simulink model "MPC_MG_freq_27072022"  (R2021b)
settings: Solver=VariableStepAuto  StartTime=0.0  StopTime=10  RelTol=1e-3
model workspace (MAT data in the model file):
  Ts : Simulink.Parameter (value not decoded)
  secondary_on : Simulink.Parameter (value not decoded)
values from neighbouring files (symbols this model uses):
  A = zeros(4,4)    [MPC_MG_script_raw_dmpc.m]    (also in MPG_MG_July.m = [0 1 1 1; 1 0 0 0; 1 0 0 0; 1 0 0 0]; MPG_MG_freq_script.m = ones(4) - eye(4); Script.m = [0 1 1 1 ; 1 0 1 1 ; 1 1 0 1 ; 1 1 1 0])
  a12 = 0    [Four_DG_MG_PrimaryOnlyScript.m]    (also in MPC_MG_script_raw_dmpc.m; MPC_MG_secondary_script.m)
  a14 = 0    [Four_DG_MG_PrimaryOnlyScript.m]    (also in MPC_MG_script_raw_dmpc.m; MPC_MG_secondary_script.m)
  a21 = 1    [Four_DG_MG_PrimaryOnlyScript.m]    (also in MPC_MG_script_raw_dmpc.m; MPC_MG_secondary_script.m)
  a23 = 0    [Four_DG_MG_PrimaryOnlyScript.m]    (also in MPC_MG_script_raw_dmpc.m; MPC_MG_secondary_script.m)
  a32 = 1    [Four_DG_MG_PrimaryOnlyScript.m]    (also in MPC_MG_script_raw_dmpc.m; MPC_MG_secondary_script.m)
  a34 = 0    [Four_DG_MG_PrimaryOnlyScript.m]    (also in MPC_MG_script_raw_dmpc.m; MPC_MG_secondary_script.m)
  a41 = 1    [Four_DG_MG_PrimaryOnlyScript.m]    (also in MPC_MG_script_raw_dmpc.m; MPC_MG_secondary_script.m)
  a43 = 0    [Four_DG_MG_PrimaryOnlyScript.m]    (also in MPC_MG_script_raw_dmpc.m; MPC_MG_secondary_script.m)
  b1v = 1    [Four_DG_MG_PrimaryOnlyScript.m]    (also in MPC_MG_script_raw_dmpc.m; MPC_MG_secondary_script.m; MPG_MG_July.m; MPG_MG_freq_script.m)
  b1w = 1    [Four_DG_MG_PrimaryOnlyScript.m]    (also in MPC_MG_script_raw_dmpc.m; MPC_MG_secondary_script.m; MPG_MG_July.m; MPG_MG_freq_script.m)
  b2v = 0    [Four_DG_MG_PrimaryOnlyScript.m]    (also in MPC_MG_script_raw_dmpc.m; MPC_MG_secondary_script.m; MPG_MG_July.m; MPG_MG_freq_script.m)
  b2w = 0    [Four_DG_MG_PrimaryOnlyScript.m]    (also in MPC_MG_script_raw_dmpc.m; MPC_MG_secondary_script.m; MPG_MG_July.m; MPG_MG_freq_script.m)
  b3v = 0    [Four_DG_MG_PrimaryOnlyScript.m]    (also in MPC_MG_script_raw_dmpc.m; MPC_MG_secondary_script.m; MPG_MG_July.m; MPG_MG_freq_script.m)
  b3w = 0    [Four_DG_MG_PrimaryOnlyScript.m]    (also in MPC_MG_script_raw_dmpc.m; MPC_MG_secondary_script.m; MPG_MG_July.m; MPG_MG_freq_script.m)
  b4v = 0    [Four_DG_MG_PrimaryOnlyScript.m]    (also in MPC_MG_script_raw_dmpc.m; MPC_MG_secondary_script.m; MPG_MG_July.m; MPG_MG_freq_script.m)
  b4w = 0    [Four_DG_MG_PrimaryOnlyScript.m]    (also in MPC_MG_script_raw_dmpc.m; MPC_MG_secondary_script.m; MPG_MG_July.m; MPG_MG_freq_script.m)
  C_f = 50e-6    (= 5e-05)    [Four_DG_MG_PrimaryOnlyScript.m]    (also in MPC_MG_script.m; MPC_MG_script_raw_dmpc.m; MPC_MG_secondary_script.m; MPG_MG_July.m)
  cf = 60    [Four_DG_MG_PrimaryOnlyScript.m]    (also in MPC_MG_script_raw_dmpc.m = 40; MPC_MG_secondary_script.m = 40; MPG_MG_July.m = 100; MPG_MG_freq_script.m = 100)
  cv = 60    [Four_DG_MG_PrimaryOnlyScript.m]    (also in MPC_MG_script_raw_dmpc.m = 40; MPC_MG_secondary_script.m = 40; MPG_MG_July.m = 100; MPG_MG_freq_script.m = 100)
  f_c = 5000    [Four_DG_MG_PrimaryOnlyScript.m]    (also in MPC_MG_script.m = 40000; MPC_MG_script_raw_dmpc.m = 40000; MPC_MG_secondary_script.m = 40000; MPG_MG_July.m = 50000)
  kL = 1e-5    (= 1e-05)    [Four_DG_MG_PrimaryOnlyScript.m]    (also in MPC_MG_script.m = 1e-08; MPC_MG_script_raw_dmpc.m = 1e-08; MPC_MG_secondary_script.m = 1e-07; MPG_MG_July.m = 1e-07)
  L_f = 1.35e-3    (= 0.00135)    [Four_DG_MG_PrimaryOnlyScript.m]    (also in MPC_MG_script.m; MPC_MG_script_raw_dmpc.m; MPC_MG_secondary_script.m; MPG_MG_July.m)
  L_in1 = 0.35e-3    (= 0.00035)    [Four_DG_MG_PrimaryOnlyScript.m]    (also in MPC_MG_script.m; MPC_MG_script_raw_dmpc.m; MPC_MG_secondary_script.m; MPG_MG_July.m)
  L_in2 = 0.35e-3    (= 0.00035)    [Four_DG_MG_PrimaryOnlyScript.m]    (also in MPC_MG_script.m; MPC_MG_script_raw_dmpc.m; MPC_MG_secondary_script.m; MPG_MG_July.m)
  L_in3 = 0.35e-3    (= 0.00035)    [Four_DG_MG_PrimaryOnlyScript.m]    (also in MPC_MG_script.m; MPC_MG_script_raw_dmpc.m; MPC_MG_secondary_script.m; MPG_MG_July.m)
  L_in4 = 0.35e-3    (= 0.00035)    [Four_DG_MG_PrimaryOnlyScript.m]    (also in MPC_MG_script.m; MPC_MG_script_raw_dmpc.m; MPC_MG_secondary_script.m; MPG_MG_July.m)
  lambda1 = [30000 50000 90000 50000]'    [MPC_MG_script_raw_dmpc.m]    (also in MPG_MG_July.m = [4 4 4 4]'; MPG_MG_freq_script.m = [3 3 3 3]'; Script.m = [1 1 1 1]')
  lambda2 = [5 6 7 6]'    [MPC_MG_script_raw_dmpc.m]    (also in MPG_MG_July.m = [0.5e-2 0.5e-2 0.5e-2 0.5e-2]'; MPG_MG_freq_script.m = [1.1 1.9 1.5 1.2]'; Script.m = [0.8e-2 0.8e-2 0.8e-2 0.8e-2]')
  lambda3 = [80000 80000 900000 80000]'    [MPC_MG_script_raw_dmpc.m]    (also in MPG_MG_July.m = [1e-3 1e-3 1e-3 1e-3]'; MPG_MG_freq_script.m = [9e-4 1.2e-2 3e-3 3e-3]'; Script.m = [1.5e-3 1.5e-3 1.5e-3 1.5e-3]')
  LD_ref1 = 800e-6    (= 0.0008)    [Four_DG_MG_PrimaryOnlyScript.m]    (also in MPC_MG_script.m = 0.0003; MPC_MG_script_raw_dmpc.m = 0.0003; MPC_MG_secondary_script.m = 0.0001; MPG_MG_July.m = 0.0004)
  lo_co = 0.2    [Four_DG_MG_PrimaryOnlyScript.m]    (also in MPC_MG_script.m = 0.05; MPC_MG_script_raw_dmpc.m; MPC_MG_secondary_script.m = 0.08; MPG_MG_July.m = 0.15)
  load_on = 3    [MPG_MG_July.m]    (also in Script.m = 1)
  m_p1 = 9.4e-5/droopDivide    (= 9.4e-05)    [Four_DG_MG_PrimaryOnlyScript.m]    (also in MPC_MG_script.m; MPC_MG_script_raw_dmpc.m; MPC_MG_secondary_script.m; MPG_MG_July.m)
  m_p2 = 9.4e-5/droopDivide    (= 9.4e-05)    [Four_DG_MG_PrimaryOnlyScript.m]    (also in MPC_MG_script.m; MPC_MG_script_raw_dmpc.m; MPC_MG_secondary_script.m; MPG_MG_July.m)
  m_p3 = 12.5e-5/droopDivide    (= 0.000125)    [Four_DG_MG_PrimaryOnlyScript.m]    (also in MPC_MG_script.m; MPC_MG_script_raw_dmpc.m; MPC_MG_secondary_script.m; MPG_MG_July.m)
  m_p4 = 12.5e-5/droopDivide    (= 0.000125)    [Four_DG_MG_PrimaryOnlyScript.m]    (also in MPC_MG_script.m; MPC_MG_script_raw_dmpc.m; MPC_MG_secondary_script.m; MPG_MG_July.m)
  N = 3    [MPG_MG_July.m]    (also in MPG_MG_freq_script.m = 2; Script.m = 5)
  n_q1 = 1.3e-3/droopDivide2    (= 0.00013)    [Four_DG_MG_PrimaryOnlyScript.m]    (also in MPC_MG_script.m; MPC_MG_script_raw_dmpc.m; MPC_MG_secondary_script.m; MPG_MG_July.m)
  n_q2 = 1.3e-3/droopDivide2    (= 0.00013)    [Four_DG_MG_PrimaryOnlyScript.m]    (also in MPC_MG_script.m; MPC_MG_script_raw_dmpc.m; MPC_MG_secondary_script.m; MPG_MG_July.m)
  n_q3 = 1.5e-3/droopDivide2    (= 0.00015)    [Four_DG_MG_PrimaryOnlyScript.m]    (also in MPC_MG_script.m; MPC_MG_script_raw_dmpc.m; MPC_MG_secondary_script.m; MPG_MG_July.m)
  n_q4 = 1.5e-3/droopDivide2    (= 0.00015)    [Four_DG_MG_PrimaryOnlyScript.m]    (also in MPC_MG_script.m; MPC_MG_script_raw_dmpc.m; MPC_MG_secondary_script.m; MPG_MG_July.m)
  Pmax = [45e3 45e3 37e3 37e3]'    [MPG_MG_July.m]    (also in MPG_MG_freq_script.m; Script.m)
  R_f = 0.1    [Four_DG_MG_PrimaryOnlyScript.m]    (also in MPC_MG_script.m; MPC_MG_script_raw_dmpc.m; MPC_MG_secondary_script.m; MPG_MG_July.m)
  R_in1 = 0.03    [Four_DG_MG_PrimaryOnlyScript.m]    (also in MPC_MG_script.m; MPC_MG_script_raw_dmpc.m; MPC_MG_secondary_script.m; MPG_MG_July.m)
  R_in2 = 0.03    [Four_DG_MG_PrimaryOnlyScript.m]    (also in MPC_MG_script.m; MPC_MG_script_raw_dmpc.m; MPC_MG_secondary_script.m; MPG_MG_July.m)
  R_in3 = 0.03    [Four_DG_MG_PrimaryOnlyScript.m]    (also in MPC_MG_script.m; MPC_MG_script_raw_dmpc.m; MPC_MG_secondary_script.m; MPG_MG_July.m)
  R_in4 = 0.03    [Four_DG_MG_PrimaryOnlyScript.m]    (also in MPC_MG_script.m; MPC_MG_script_raw_dmpc.m; MPC_MG_secondary_script.m; MPG_MG_July.m)
  time_thresh = 0.6    [Four_DG_MG_PrimaryOnlyScript.m]    (also in MPC_MG_script_raw_dmpc.m = 1.5; MPC_MG_secondary_script.m = 2; MPG_MG_July.m = 0.5; MPG_MG_freq_script.m = 0.5)
  Ts = 10e-6    (= 1e-05)    [Four_DG_MG_PrimaryOnlyScript.m]    (also in MPC_MG_script.m; MPC_MG_script_raw_dmpc.m; MPC_MG_secondary_script.m; MPG_MG_July.m)
  Tsamp = 0.1    [MPG_MG_July.m]    (also in MPG_MG_freq_script.m; Script.m)
  V_nom = 220*sqrt(2)    [Four_DG_MG_PrimaryOnlyScript.m]    (also in MPC_MG_script.m; MPC_MG_script_raw_dmpc.m; MPC_MG_secondary_script.m; MPG_MG_July.m)
  Vdc = 600    [Four_DG_MG_PrimaryOnlyScript.m]    (also in MPC_MG_script.m; MPC_MG_script_raw_dmpc.m; MPC_MG_secondary_script.m; MPG_MG_July.m)
  w_c_high = 2*pi*50    (= 314.159265359)    [Four_DG_MG_PrimaryOnlyScript.m]    (also in MPC_MG_script.m; MPC_MG_script_raw_dmpc.m; MPC_MG_secondary_script.m; MPG_MG_July.m)
  w_nom = 2*pi*50    (= 314.159265359)    [Four_DG_MG_PrimaryOnlyScript.m]    (also in MPC_MG_script.m; MPC_MG_script_raw_dmpc.m; MPC_MG_secondary_script.m; MPG_MG_July.m)
undefined symbols (not defined in the file or in its folder): a13, a24, a31, a42, DiscIntNeverNeededParam, i
libraries: eeGeneralControl x29, spsThreePhaseSeriesRLCBranchLib x24, spsThreePhaseVIMeasurementLib x21, spsabctodq0Lib x16, slpidlib x12, spsDCVoltageSourceLib x7, spsSeriesRLCBranchLib x7, spsTwoLevelConverterLib x7, spsGroundLib x6, spsThreePhaseSeriesRLCLoadLib x5, dspswit3 x5, spsThreePhaseBreakerLib x4
(part 3 of 7)

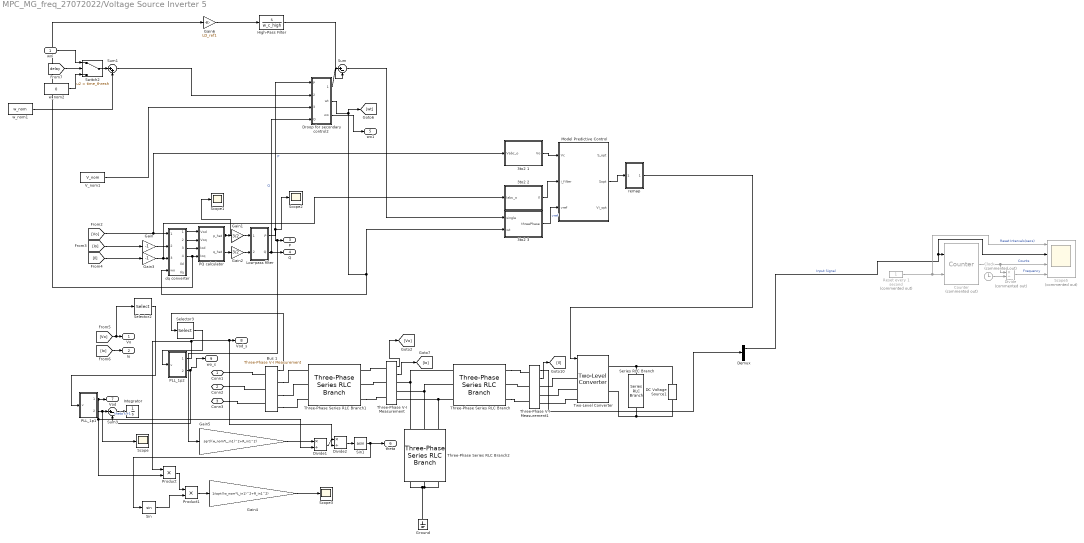
== system MPC_MG_freq_27072022/Voltage Source Inverter 5 ==
  wni : Inport
  3to2 1 : Subsystem
  3to2 2 : Subsystem
  3to2 3 : Subsystem
  Bus 1 : spsThreePhaseVIMeasurementLib/Three-Phase V-I Measurement  VoltageMeasurement=phase-to-ground  SetLabelV=off  LabelV=Vbus  Vpu=off  VpuLL=off  CurrentMeasurement=no  SetLabelI=off  LabelI=Ibus  Ipu=off  Pbase=100e6  Vbase=380  OutputType=Complex  PhasorSimulation=off  PSBequivalent=0
  Clock : Clock  Commented=on
  Counter : dspswit3/Counter  Commented=on  Direction=Up  CountEvent=Rising edge  CounterSize=User defined  MaxCount=5e5  InitialCount=0  Output=Count  HitValue=1  ResetInput=on  SamplesPerFrame=1  Ts=1  CntDtype=double  HitDtype=Logical
  DC Voltage Source1 : spsDCVoltageSourceLib/DC Voltage Source  Amplitude=Vdc  Measurements=None
  Demux : Demux  Outputs=3
  Divide : Product  Commented=on  Inputs=*/
  Divide1 : Product  Inputs=*/
  Divide2 : Product  Inputs=*/
  Droop for secondary control2 : Subsystem
  Gain : Gain  Gain=-1
  Gain1 : Gain  Gain=3/2
  Gain2 : Gain  Gain=3/2
  Gain3 : Gain  Gain=-1
  Gain4 : Gain  Gain=1/sqrt((w_nom*L_in1)^2+R_in1^2)
  Gain5 : Gain  Gain=sqrt((w_nom*L_in1)^2+R_in1^2)
  Gain6 : Gain  Gain=LD_ref1
  Ground : spsGroundLib/Ground  LConnTagsString=a
  High-Pass Filter : TransferFcn  Numerator=[1 0]  Denominator=w_c_high
  Integrator : Integrator
  Low-pass filter : Subsystem
  "Model Predictive Control " : MATLAB Function  TreatAsAtomicUnit=on  mask{Ts=modT, Cfilter=C_f, Lfilter=L_f, Vdc=Vdc}
      mask prompts: Ts "Sampling Time"; Cfilter "Filter Capacitor"; Lfilter "Filter Inductance"; Vdc "Input DC Voltage"
  PLL_1p1 : Subsystem  SystemSampleTime=10*Ts
      settings: MinAlgLoopOccurrences=on
  PLL_1p2 : Subsystem  SystemSampleTime=10*Ts
      settings: MinAlgLoopOccurrences=on
  PQ calculator : Subsystem
  Product : Product
  Product1 : Product
  Reset every 1 second : Constant  Commented=on
  Scope{,1..3} (4 alike) : Scope
  Scope5 : Scope  Commented=on  NumInputPorts=4
  Selector2 : Selector  InputPortWidth=3  IndexOptions=Index vector (dialog)  Indices=[1]  OutputSizes=1
  Selector3 : Selector  InputPortWidth=3  IndexOptions=Index vector (dialog)  Indices=[1]  OutputSizes=1
  Series RLC Branch : spsSeriesRLCBranchLib/Series RLC Branch  LConnTagsString=__new0  RConnTagsString=__new0  BranchType=RC  Resistance=30  Inductance=1e-3  SetiL0=off  InitialCurrent=0  Capacitance=80e-6  Setx0=off  InitialVoltage=0  Measurements=None
  Sin : Trigonometry
  Sin1 : Trigonometry  Operator=asin
  Sum : Sum  Inputs=|+-
  Sum1 : Sum  Inputs=|++
  Sum3 : Sum  Inputs=|+-
  Switch2 : Switch  Criteria=u2 > Threshold  Threshold=time_thresh
  Three-Phase Series RLC Branch : spsThreePhaseSeriesRLCBranchLib/Three-Phase Series RLC Branch  LConnTagsString=A|B|C  RConnTagsString=A|B|C  BranchType=RL  Resistance=R_f  Inductance=L_f  Capacitance=1e-6  Measurements=None
  Three-Phase Series RLC Branch1 : spsThreePhaseSeriesRLCBranchLib/Three-Phase Series RLC Branch  LConnTagsString=A|B|C  RConnTagsString=A|B|C  BranchType=RL  Resistance=R_in  Inductance=L_in  Capacitance=1e-6  Measurements=None
  Three-Phase Series RLC Branch2 : spsThreePhaseSeriesRLCBranchLib/Three-Phase Series RLC Branch  LConnTagsString=A|B|C  RConnTagsString=A|B|C  BranchType=C  Resistance=R_f  Inductance=1e-3  Capacitance=C_f  Measurements=None
  Three-Phase V-I Measurement : spsThreePhaseVIMeasurementLib/Three-Phase V-I Measurement  VoltageMeasurement=phase-to-ground  SetLabelV=off  LabelV=Vo1  Vpu=off  VpuLL=off  CurrentMeasurement=yes  SetLabelI=off  LabelI=Io1  Ipu=off  Pbase=100e6  Vbase=500e3  OutputType=Complex  PhasorSimulation=off  PSBequivalent=0
  Three-Phase V-I Measurement1 : spsThreePhaseVIMeasurementLib/Three-Phase V-I Measurement  VoltageMeasurement=phase-to-ground  SetLabelV=off  LabelV=Vl2  Vpu=off  VpuLL=off  CurrentMeasurement=yes  SetLabelI=off  LabelI=Il2  Ipu=off  Pbase=100e6  Vbase=500e3  OutputType=Complex  PhasorSimulation=off  PSBequivalent=0
  Two-Level Converter : spsTwoLevelConverterLib/Two-Level Converter  ModelType=Switching devices  Ron=1e-3  Rs=1e6  Cs=inf  Vforward=[0,0]  Ron_Diode=1e-3  Rs_Diode=1e6  Cs_Diode=inf  Vf_Diode=1e-3  Rs_CurrentSource=inf
      settings: SourceProductBaseCode=PS
  V_nom1 : Constant  Value=V_nom
  dq converter : Subsystem
  remap : Subsystem
  w_nom1 : Constant  Value=w_nom
  w_nom2 : Constant  Value=0
  Conn1 : PMIOPort  Side=Left
  Conn2 : PMIOPort  Port=2  Side=Left
  Conn3 : PMIOPort  Port=3  Side=Left
  Vo : Outport
  Io : Outport  Port=2
  P : Outport  Port=3
  Q : Outport  Port=4
  wo1 : Outport  Port=5
  theta : Outport  Port=6
  Vod : Outport  Port=7
  Vod_s : Outport  Port=8
  wo_s : Outport  Port=9
  wires:
  Gain/1 -> dq converter/2(Iodq)
  Gain2/1 -> Low-pass filter/2(q_hat)
  PQ calculator/2(q_hat) -> Gain2/1
  Gain1/1 -> Low-pass filter/1(p_hat)
  PQ calculator/1(p_hat) -> Scope1/1, Gain1/1
  [Vo] -> Selector2/1, Vo/1
  [Io] -> Io/1
  Three-Phase V-I Measurement/1 -> [Vo]
  Three-Phase V-I Measurement/2 -> [Io]
  Three-Phase V-I Measurement1/2 -> [Il]
  3to2 1/1(Vo) -> "Model Predictive Control "/1(Vc)
  3to2 3/1(threePhase) -> "Model Predictive Control "/3(vref)  "vref"
  3to2 2/1(Il) -> "Model Predictive Control "/2(i_filter)
  "Model Predictive Control "/2(Sopt) -> remap/1(In1)
  Gain3/1 -> dq converter/3(Ildq), 3to2 2/1("Iabc_o ")
  remap/1(Out1) -> Two-Level Converter/1
  [Vo] -> dq converter/1(Vodq), 3to2 1/1("Vabc_o ")
  [Io] -> Gain/1
  [Il] -> Gain3/1
  Sum/1 -> 3to2 3/1("single ")
  Three-Phase V-I Measurement1/1 -> Demux/1
  Demux/1 -> Counter/1, Scope5/2  "Input Signal"
  Clock/1 -> Divide/2
  Reset every 1 second/1 -> Scope5/1, Counter/2  "Reset Intervals(secs)"
  Counter/1 -> Scope5/3, Divide/1  "Counts"
  Divide/1 -> Scope5/4  "Frequency"
  dq converter/4(Ioq) -> Gain6/1, PQ calculator/4(Ioq)
  Low-pass filter/2(Q) -> Q/1, Droop for secondary control2/4(Q)  "Q"
  dq converter/3(Iod) -> PQ calculator/3(Iod)
  Low-pass filter/1(P) -> Scope2/1, Gain5/1, P/1, Droop for secondary control2/1(P)  "P"
  Sum1/1 -> Droop for secondary control2/2(w_nom)
  V_nom1/1 -> Droop for secondary control2/3(V_nom)
  Selector2/1 -> PLL_1p1/1(v)
  Selector3/1 -> PLL_1p2/1(v)
  PLL_1p2/1(v_dq) -> Product/1, Divide2/2, Vod_s/1
  Droop for secondary control2/1(Vref) -> Sum/1
  High-Pass Filter/1 -> Sum/2
  Gain6/1 -> High-Pass Filter/1
  [delay] -> Switch2/2
  Switch2/1 -> Sum1/1
  w_nom2/1 -> Switch2/3
  w_nom1/1 -> Sum1/2
  wni/1 -> Switch2/1
  dq converter/2(Voq) -> PQ calculator/2(Voq)
  dq converter/1(Vod) -> PQ calculator/1(Vod)
  PLL_1p2/2(omega) -> Sum3/2, wo_s/1
  Bus 1/1 -> Selector3/1
  Droop for secondary control2/2(wt) -> [wt], dq converter/4(wo), 3to2 3/2("wt ")
  Droop for secondary control2/3(wo) -> wo1/1
  PLL_1p1/2(omega) -> Scope/1, Sum3/1
  PLL_1p1/1(v_dq) -> Product/2, Divide1/2, Vod/1
  Sum3/1 -> Integrator/1  "theta k+1"
  Gain5/1 -> Divide1/1
  Divide1/1 -> Divide2/1
  Divide2/1 -> Sin1/1
  Sin1/1 -> Sin/1, theta/1
  Product1/1 -> Gain4/1
  Product/1 -> Product1/1
  Sin/1 -> Product1/2
  Gain4/1 -> Scope3/1
  connections:
  Three-Phase Series RLC Branch2/LConn1 -- Three-Phase V-I Measurement/RConn1 -- Three-Phase Series RLC Branch/LConn1
  Two-Level Converter/RConn1 -- DC Voltage Source1/RConn1 -- Series RLC Branch/LConn1
  Three-Phase Series RLC Branch2/RConn3 -- Ground/LConn1 -- Three-Phase Series RLC Branch2/RConn1 -- Three-Phase Series RLC Branch2/RConn2
  Three-Phase Series RLC Branch2/LConn3 -- Three-Phase Series RLC Branch/LConn3 -- Three-Phase V-I Measurement/RConn3
  Two-Level Converter/RConn2 -- Series RLC Branch/RConn1 -- DC Voltage Source1/LConn1
  Three-Phase Series RLC Branch/LConn2 -- Three-Phase V-I Measurement/RConn2 -- Three-Phase Series RLC Branch2/LConn2
  Two-Level Converter/LConn1 -- Three-Phase V-I Measurement1/RConn1
  Three-Phase V-I Measurement1/LConn2 -- Three-Phase Series RLC Branch/RConn2
  Two-Level Converter/LConn2 -- Three-Phase V-I Measurement1/RConn2
  Two-Level Converter/LConn3 -- Three-Phase V-I Measurement1/RConn3
  Three-Phase Series RLC Branch/RConn1 -- Three-Phase V-I Measurement1/LConn1
  Three-Phase V-I Measurement/LConn1 -- Three-Phase Series RLC Branch1/RConn1
  Three-Phase V-I Measurement/LConn2 -- Three-Phase Series RLC Branch1/RConn2
  Three-Phase Series RLC Branch1/RConn3 -- Three-Phase V-I Measurement/LConn3
  Three-Phase Series RLC Branch/RConn3 -- Three-Phase V-I Measurement1/LConn3
  Conn1/RConn1 -- Bus 1/LConn1
  Conn2/RConn1 -- Bus 1/LConn2
  Conn3/RConn1 -- Bus 1/LConn3
  Bus 1/RConn1 -- Three-Phase Series RLC Branch1/LConn1
  Bus 1/RConn2 -- Three-Phase Series RLC Branch1/LConn2
  Bus 1/RConn3 -- Three-Phase Series RLC Branch1/LConn3

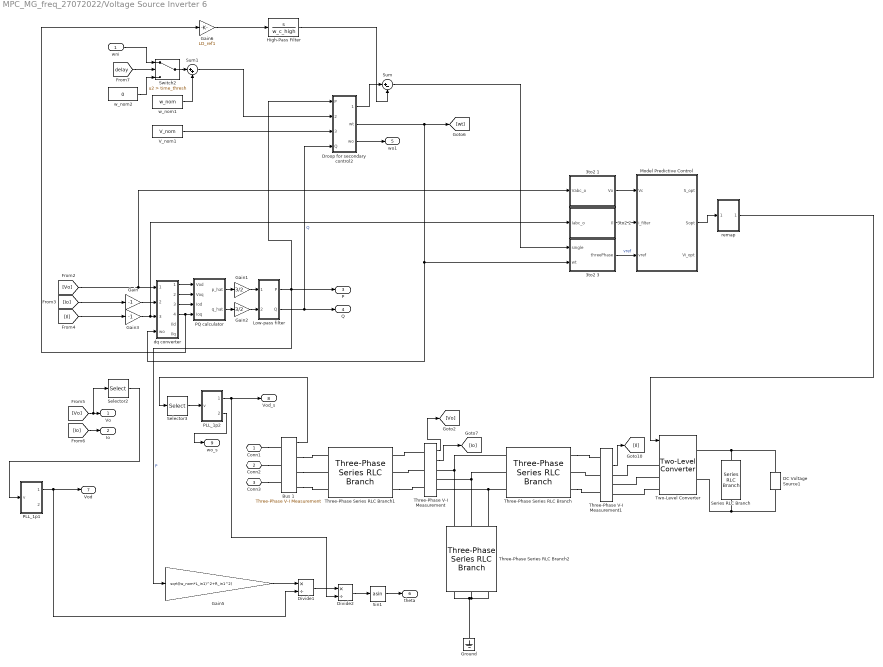
== system MPC_MG_freq_27072022/Voltage Source Inverter 6 ==
  wni : Inport
  3to2 1 : Subsystem
  3to2 2 : Subsystem
  3to2 3 : Subsystem
  Bus 1 : spsThreePhaseVIMeasurementLib/Three-Phase V-I Measurement  VoltageMeasurement=phase-to-ground  SetLabelV=off  LabelV=Vbus  Vpu=off  VpuLL=off  CurrentMeasurement=no  SetLabelI=off  LabelI=Ibus  Ipu=off  Pbase=100e6  Vbase=380  OutputType=Complex  PhasorSimulation=off  PSBequivalent=0
  DC Voltage Source1 : spsDCVoltageSourceLib/DC Voltage Source  Amplitude=Vdc  Measurements=None
  Divide1 : Product  Inputs=*/
  Divide2 : Product  Inputs=*/
  Droop for secondary control2 : Subsystem
  Gain : Gain  Gain=-1
  Gain1 : Gain  Gain=3/2
  Gain2 : Gain  Gain=3/2
  Gain3 : Gain  Gain=-1
  Gain5 : Gain  Gain=sqrt((w_nom*L_in1)^2+R_in1^2)
  Gain6 : Gain  Gain=LD_ref1
  Ground : spsGroundLib/Ground  LConnTagsString=a
  High-Pass Filter : TransferFcn  Numerator=[1 0]  Denominator=w_c_high
  Low-pass filter : Subsystem
  "Model Predictive Control " : MATLAB Function  TreatAsAtomicUnit=on  mask{Ts=modT, Cfilter=C_f, Lfilter=L_f, Vdc=Vdc}
      mask prompts: Ts "Sampling Time"; Cfilter "Filter Capacitor"; Lfilter "Filter Inductance"; Vdc "Input DC Voltage"
  PLL_1p1 : Subsystem  SystemSampleTime=10*Ts
      settings: MinAlgLoopOccurrences=on
  PLL_1p2 : Subsystem  SystemSampleTime=10*Ts
      settings: MinAlgLoopOccurrences=on
  PQ calculator : Subsystem
  Selector2 : Selector  InputPortWidth=3  IndexOptions=Index vector (dialog)  Indices=[1]  OutputSizes=1
  Selector3 : Selector  InputPortWidth=3  IndexOptions=Index vector (dialog)  Indices=[1]  OutputSizes=1
  Series RLC Branch : spsSeriesRLCBranchLib/Series RLC Branch  LConnTagsString=__new0  RConnTagsString=__new0  BranchType=RC  Resistance=30  Inductance=1e-3  SetiL0=off  InitialCurrent=0  Capacitance=80e-6  Setx0=off  InitialVoltage=0  Measurements=None
  Sin1 : Trigonometry  Operator=asin
  Sum : Sum  Inputs=|+-
  Sum1 : Sum  Inputs=|++
  Switch2 : Switch  Criteria=u2 > Threshold  Threshold=time_thresh
  Three-Phase Series RLC Branch : spsThreePhaseSeriesRLCBranchLib/Three-Phase Series RLC Branch  LConnTagsString=A|B|C  RConnTagsString=A|B|C  BranchType=RL  Resistance=R_f  Inductance=L_f  Capacitance=1e-6  Measurements=None
  Three-Phase Series RLC Branch1 : spsThreePhaseSeriesRLCBranchLib/Three-Phase Series RLC Branch  LConnTagsString=A|B|C  RConnTagsString=A|B|C  BranchType=RL  Resistance=R_in  Inductance=L_in  Capacitance=1e-6  Measurements=None
  Three-Phase Series RLC Branch2 : spsThreePhaseSeriesRLCBranchLib/Three-Phase Series RLC Branch  LConnTagsString=A|B|C  RConnTagsString=A|B|C  BranchType=C  Resistance=R_f  Inductance=1e-3  Capacitance=C_f  Measurements=None
  Three-Phase V-I Measurement : spsThreePhaseVIMeasurementLib/Three-Phase V-I Measurement  VoltageMeasurement=phase-to-ground  SetLabelV=off  LabelV=Vo1  Vpu=off  VpuLL=off  CurrentMeasurement=yes  SetLabelI=off  LabelI=Io1  Ipu=off  Pbase=100e6  Vbase=500e3  OutputType=Complex  PhasorSimulation=off  PSBequivalent=0
  Three-Phase V-I Measurement1 : spsThreePhaseVIMeasurementLib/Three-Phase V-I Measurement  VoltageMeasurement=phase-to-ground  SetLabelV=off  LabelV=Vl2  Vpu=off  VpuLL=off  CurrentMeasurement=yes  SetLabelI=off  LabelI=Il2  Ipu=off  Pbase=100e6  Vbase=500e3  OutputType=Complex  PhasorSimulation=off  PSBequivalent=0
  Two-Level Converter : spsTwoLevelConverterLib/Two-Level Converter  ModelType=Switching devices  Ron=1e-3  Rs=1e6  Cs=inf  Vforward=[0,0]  Ron_Diode=1e-3  Rs_Diode=1e6  Cs_Diode=inf  Vf_Diode=1e-3  Rs_CurrentSource=inf
      settings: SourceProductBaseCode=PS
  V_nom1 : Constant  Value=V_nom
  dq converter : Subsystem
  remap : Subsystem
  w_nom1 : Constant  Value=w_nom
  w_nom2 : Constant  Value=0
  Conn1 : PMIOPort  Side=Left
  Conn2 : PMIOPort  Port=2  Side=Left
  Conn3 : PMIOPort  Port=3  Side=Left
  Vo : Outport
  Io : Outport  Port=2
  P : Outport  Port=3
  Q : Outport  Port=4
  wo1 : Outport  Port=5
  theta : Outport  Port=6
  Vod : Outport  Port=7
  Vod_s : Outport  Port=8
  wo_s : Outport  Port=9
  wires:
  Gain/1 -> dq converter/2(Iodq)
  Gain2/1 -> Low-pass filter/2(q_hat)
  PQ calculator/2(q_hat) -> Gain2/1
  Gain1/1 -> Low-pass filter/1(p_hat)
  PQ calculator/1(p_hat) -> Gain1/1
  [Vo] -> Selector2/1, Vo/1
  [Io] -> Io/1
  Three-Phase V-I Measurement/1 -> [Vo]
  Three-Phase V-I Measurement/2 -> [Io]
  Three-Phase V-I Measurement1/2 -> [Il]
  3to2 1/1(Vo) -> "Model Predictive Control "/1(Vc)
  3to2 3/1(threePhase) -> "Model Predictive Control "/3(vref)  "vref"
  3to2 2/1(Il) -> "Model Predictive Control "/2(i_filter)
  "Model Predictive Control "/2(Sopt) -> remap/1(In1)
  Gain3/1 -> dq converter/3(Ildq), 3to2 2/1("Iabc_o ")
  remap/1(Out1) -> Two-Level Converter/1
  [Vo] -> dq converter/1(Vodq), 3to2 1/1("Vabc_o ")
  [Io] -> Gain/1
  [Il] -> Gain3/1
  Sum/1 -> 3to2 3/1("single ")
  dq converter/4(Ioq) -> Gain6/1, PQ calculator/4(Ioq)
  Low-pass filter/2(Q) -> Droop for secondary control2/4(Q), Q/1  "Q"
  dq converter/3(Iod) -> PQ calculator/3(Iod)
  Low-pass filter/1(P) -> Droop for secondary control2/1(P), Gain5/1, P/1  "P"
  Sum1/1 -> Droop for secondary control2/2(w_nom)
  V_nom1/1 -> Droop for secondary control2/3(V_nom)
  Selector2/1 -> PLL_1p1/1(v)
  Selector3/1 -> PLL_1p2/1(v)
  PLL_1p2/1(v_dq) -> Divide2/2, Vod_s/1
  Droop for secondary control2/1(Vref) -> Sum/1
  High-Pass Filter/1 -> Sum/2
  Gain6/1 -> High-Pass Filter/1
  [delay] -> Switch2/2
  Switch2/1 -> Sum1/1
  w_nom2/1 -> Switch2/3
  w_nom1/1 -> Sum1/2
  wni/1 -> Switch2/1
  dq converter/2(Voq) -> PQ calculator/2(Voq)
  dq converter/1(Vod) -> PQ calculator/1(Vod)
  PLL_1p2/2(omega) -> wo_s/1
  Bus 1/1 -> Selector3/1
  Droop for secondary control2/2(wt) -> dq converter/4(wo), 3to2 3/2("wt "), [wt]
  Droop for secondary control2/3(wo) -> wo1/1
  PLL_1p1/1(v_dq) -> Vod/1, Divide1/2
  Gain5/1 -> Divide1/1
  Divide1/1 -> Divide2/1
  Divide2/1 -> Sin1/1
  Sin1/1 -> theta/1
  connections:
  Three-Phase Series RLC Branch2/LConn1 -- Three-Phase V-I Measurement/RConn1 -- Three-Phase Series RLC Branch/LConn1
  Two-Level Converter/RConn1 -- DC Voltage Source1/RConn1 -- Series RLC Branch/LConn1
  Three-Phase Series RLC Branch2/RConn3 -- Ground/LConn1 -- Three-Phase Series RLC Branch2/RConn1 -- Three-Phase Series RLC Branch2/RConn2
  Three-Phase Series RLC Branch2/LConn3 -- Three-Phase Series RLC Branch/LConn3 -- Three-Phase V-I Measurement/RConn3
  Two-Level Converter/RConn2 -- Series RLC Branch/RConn1 -- DC Voltage Source1/LConn1
  Three-Phase Series RLC Branch/LConn2 -- Three-Phase V-I Measurement/RConn2 -- Three-Phase Series RLC Branch2/LConn2
  Two-Level Converter/LConn1 -- Three-Phase V-I Measurement1/RConn1
  Three-Phase V-I Measurement1/LConn2 -- Three-Phase Series RLC Branch/RConn2
  Two-Level Converter/LConn2 -- Three-Phase V-I Measurement1/RConn2
  Two-Level Converter/LConn3 -- Three-Phase V-I Measurement1/RConn3
  Three-Phase Series RLC Branch/RConn1 -- Three-Phase V-I Measurement1/LConn1
  Three-Phase V-I Measurement/LConn1 -- Three-Phase Series RLC Branch1/RConn1
  Three-Phase V-I Measurement/LConn2 -- Three-Phase Series RLC Branch1/RConn2
  Three-Phase Series RLC Branch1/RConn3 -- Three-Phase V-I Measurement/LConn3
  Three-Phase Series RLC Branch/RConn3 -- Three-Phase V-I Measurement1/LConn3
  Conn1/RConn1 -- Bus 1/LConn1
  Conn2/RConn1 -- Bus 1/LConn2
  Conn3/RConn1 -- Bus 1/LConn3
  Bus 1/RConn1 -- Three-Phase Series RLC Branch1/LConn1
  Bus 1/RConn2 -- Three-Phase Series RLC Branch1/LConn2
  Bus 1/RConn3 -- Three-Phase Series RLC Branch1/LConn3

== system MPC_MG_freq_27072022/MPC-based Secondary Controller1/Subsystem ==
  In1 : Inport
  In2 : Inport  Port=2
  In3 : Inport  Port=3
  In4 : Inport  Port=4
  In5 : Inport  Port=5
  In6 : Inport  Port=6
  Demux : Demux  Outputs=6
  Mux : Mux  Inputs=6
  Rate Transition : RateTransition  InitialCondition=10e-6  OutPortSampleTime=Tsamp
  Out1 : Outport
  Out2 : Outport  Port=2
  Out3 : Outport  Port=3
  Out4 : Outport  Port=4
  Out5 : Outport  Port=5
  Out6 : Outport  Port=6
  wires:
  In6/1 -> Mux/6
  Mux/1 -> Rate Transition/1
  Demux/5 -> Out5/1
  Rate Transition/1 -> Demux/1
  In5/1 -> Mux/5
  Demux/3 -> Out3/1
  In3/1 -> Mux/3
  Demux/4 -> Out4/1
  In4/1 -> Mux/4
  Demux/2 -> Out2/1
  Demux/1 -> Out1/1
  Demux/6 -> Out6/1
  In2/1 -> Mux/2
  In1/1 -> Mux/1

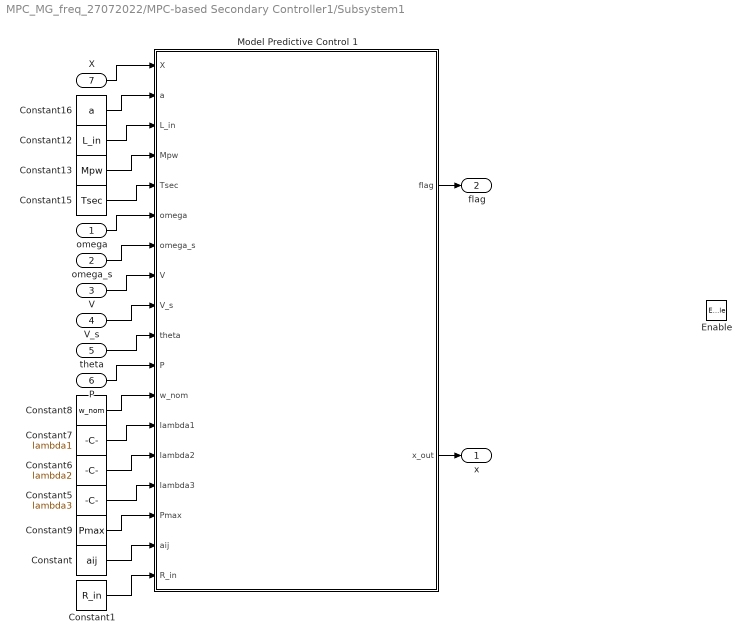
== system MPC_MG_freq_27072022/MPC-based Secondary Controller1/Subsystem1 ==
  omega : Inport
  omega_s : Inport  Port=2
  V : Inport  Port=3
  V_s : Inport  Port=4
  theta : Inport  Port=5
  P : Inport  Port=6
  X : Inport  Port=7
  Enable : EnablePort
  Constant : Constant  Value=aij
  Constant1 : Constant  Value=R_in
  Constant12 : Constant  Value=L_in
  Constant13 : Constant  Value=Mpw
  Constant15 : Constant  Value=Tsec
  Constant16 : Constant  Value=a
  Constant5 : Constant  Value=lambda3
  Constant6 : Constant  Value=lambda2
  Constant7 : Constant  Value=lambda1
  Constant8 : Constant  Value=w_nom
  Constant9 : Constant  Value=Pmax
  Model Predictive Control 1 : MATLAB Function  SystemSampleTime=Tsamp
      settings: MinAlgLoopOccurrences=on
  x : Outport
  flag : Outport  Port=2
  wires:
  Constant8/1 -> Model Predictive Control 1/12(w_nom)
  V_s/1 -> Model Predictive Control 1/9(V_s)
  P/1 -> Model Predictive Control 1/11(P)
  omega_s/1 -> Model Predictive Control 1/7(omega_s)
  Constant/1 -> Model Predictive Control 1/17(aij)
  Constant15/1 -> Model Predictive Control 1/5(Tsec)
  omega/1 -> Model Predictive Control 1/6(omega)
  Model Predictive Control 1/2(x_out) -> x/1
  Constant16/1 -> Model Predictive Control 1/2(a)
  Constant13/1 -> Model Predictive Control 1/4(Mpw)
  X/1 -> Model Predictive Control 1/1(X)
  Constant12/1 -> Model Predictive Control 1/3(L_in)
  Constant9/1 -> Model Predictive Control 1/16(Pmax)
  Constant7/1 -> Model Predictive Control 1/13(lambda1)
  Constant5/1 -> Model Predictive Control 1/15(lambda3)
  V/1 -> Model Predictive Control 1/8(V)
  theta/1 -> Model Predictive Control 1/10(theta)
  Constant6/1 -> Model Predictive Control 1/14(lambda2)
  Model Predictive Control 1/1(flag) -> flag/1
  Constant1/1 -> Model Predictive Control 1/18(R_in)

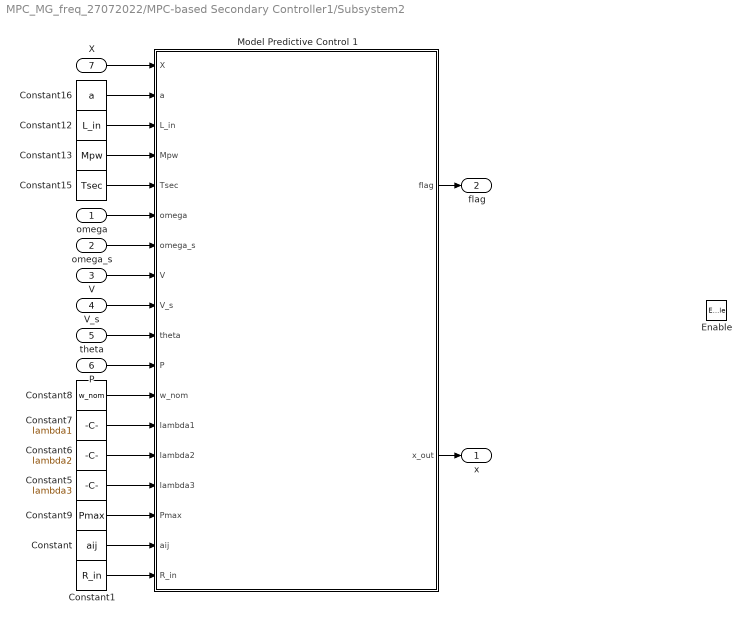
== system MPC_MG_freq_27072022/MPC-based Secondary Controller1/Subsystem2 ==
  omega : Inport
  omega_s : Inport  Port=2
  V : Inport  Port=3
  V_s : Inport  Port=4
  theta : Inport  Port=5
  P : Inport  Port=6
  X : Inport  Port=7
  Enable : EnablePort
  Constant : Constant  Value=aij
  Constant1 : Constant  Value=R_in
  Constant12 : Constant  Value=L_in
  Constant13 : Constant  Value=Mpw
  Constant15 : Constant  Value=Tsec
  Constant16 : Constant  Value=a
  Constant5 : Constant  Value=lambda3
  Constant6 : Constant  Value=lambda2
  Constant7 : Constant  Value=lambda1
  Constant8 : Constant  Value=w_nom
  Constant9 : Constant  Value=Pmax
  Model Predictive Control 1 : MATLAB Function  SystemSampleTime=Tsamp
      settings: MinAlgLoopOccurrences=on
  x : Outport
  flag : Outport  Port=2
  wires:
  Constant8/1 -> Model Predictive Control 1/12(w_nom)
  V_s/1 -> Model Predictive Control 1/9(V_s)
  P/1 -> Model Predictive Control 1/11(P)
  omega_s/1 -> Model Predictive Control 1/7(omega_s)
  Constant/1 -> Model Predictive Control 1/17(aij)
  Constant15/1 -> Model Predictive Control 1/5(Tsec)
  omega/1 -> Model Predictive Control 1/6(omega)
  Model Predictive Control 1/2(x_out) -> x/1
  Constant16/1 -> Model Predictive Control 1/2(a)
  Constant13/1 -> Model Predictive Control 1/4(Mpw)
  X/1 -> Model Predictive Control 1/1(X)
  Constant12/1 -> Model Predictive Control 1/3(L_in)
  Constant9/1 -> Model Predictive Control 1/16(Pmax)
  Constant7/1 -> Model Predictive Control 1/13(lambda1)
  Constant5/1 -> Model Predictive Control 1/15(lambda3)
  V/1 -> Model Predictive Control 1/8(V)
  theta/1 -> Model Predictive Control 1/10(theta)
  Constant6/1 -> Model Predictive Control 1/14(lambda2)
  Model Predictive Control 1/1(flag) -> flag/1
  Constant1/1 -> Model Predictive Control 1/18(R_in)

== system MPC_MG_freq_27072022/MPC-based Secondary Controller1/Subsystem3 ==
  omega : Inport
  omega_s : Inport  Port=2
  V : Inport  Port=3
  V_s : Inport  Port=4
  theta : Inport  Port=5
  P : Inport  Port=6
  X : Inport  Port=7
  Enable : EnablePort
  Constant : Constant  Value=aij
  Constant1 : Constant  Value=R_in
  Constant12 : Constant  Value=L_in
  Constant13 : Constant  Value=Mpw
  Constant15 : Constant  Value=Tsec
  Constant16 : Constant  Value=a
  Constant5 : Constant  Value=lambda3
  Constant6 : Constant  Value=lambda2
  Constant7 : Constant  Value=lambda1
  Constant8 : Constant  Value=w_nom
  Constant9 : Constant  Value=Pmax
  Model Predictive Control 1 : MATLAB Function  SystemSampleTime=Tsamp
      settings: MinAlgLoopOccurrences=on
  x : Outport
  flag : Outport  Port=2
  wires:
  Constant8/1 -> Model Predictive Control 1/12(w_nom)
  V_s/1 -> Model Predictive Control 1/9(V_s)
  P/1 -> Model Predictive Control 1/11(P)
  omega_s/1 -> Model Predictive Control 1/7(omega_s)
  Constant/1 -> Model Predictive Control 1/17(aij)
  Constant15/1 -> Model Predictive Control 1/5(Tsec)
  omega/1 -> Model Predictive Control 1/6(omega)
  Model Predictive Control 1/2(x_out) -> x/1
  Constant16/1 -> Model Predictive Control 1/2(a)
  Constant13/1 -> Model Predictive Control 1/4(Mpw)
  X/1 -> Model Predictive Control 1/1(X)
  Constant12/1 -> Model Predictive Control 1/3(L_in)
  Constant9/1 -> Model Predictive Control 1/16(Pmax)
  Constant7/1 -> Model Predictive Control 1/13(lambda1)
  Constant5/1 -> Model Predictive Control 1/15(lambda3)
  V/1 -> Model Predictive Control 1/8(V)
  theta/1 -> Model Predictive Control 1/10(theta)
  Constant6/1 -> Model Predictive Control 1/14(lambda2)
  Model Predictive Control 1/1(flag) -> flag/1
  Constant1/1 -> Model Predictive Control 1/18(R_in)

== system MPC_MG_freq_27072022/MPC-based Secondary Controller1/Subsystem4 ==
  omega : Inport
  omega_s : Inport  Port=2
  V : Inport  Port=3
  V_s : Inport  Port=4
  theta : Inport  Port=5
  P : Inport  Port=6
  X : Inport  Port=7
  Enable : EnablePort
  Constant : Constant  Value=aij
  Constant1 : Constant  Value=R_in
  Constant12 : Constant  Value=L_in
  Constant13 : Constant  Value=Mpw
  Constant15 : Constant  Value=Tsec
  Constant16 : Constant  Value=a
  Constant5 : Constant  Value=lambda3
  Constant6 : Constant  Value=lambda2
  Constant7 : Constant  Value=lambda1
  Constant8 : Constant  Value=w_nom
  Constant9 : Constant  Value=Pmax
  Model Predictive Control 1 : MATLAB Function  SystemSampleTime=Tsamp
      settings: MinAlgLoopOccurrences=on
  x : Outport
  flag : Outport  Port=2
  wires:
  Constant8/1 -> Model Predictive Control 1/12(w_nom)
  V_s/1 -> Model Predictive Control 1/9(V_s)
  P/1 -> Model Predictive Control 1/11(P)
  omega_s/1 -> Model Predictive Control 1/7(omega_s)
  Constant/1 -> Model Predictive Control 1/17(aij)
  Constant15/1 -> Model Predictive Control 1/5(Tsec)
  omega/1 -> Model Predictive Control 1/6(omega)
  Model Predictive Control 1/2(x_out) -> x/1
  Constant16/1 -> Model Predictive Control 1/2(a)
  Constant13/1 -> Model Predictive Control 1/4(Mpw)
  X/1 -> Model Predictive Control 1/1(X)
  Constant12/1 -> Model Predictive Control 1/3(L_in)
  Constant9/1 -> Model Predictive Control 1/16(Pmax)
  Constant7/1 -> Model Predictive Control 1/13(lambda1)
  Constant5/1 -> Model Predictive Control 1/15(lambda3)
  V/1 -> Model Predictive Control 1/8(V)
  theta/1 -> Model Predictive Control 1/10(theta)
  Constant6/1 -> Model Predictive Control 1/14(lambda2)
  Model Predictive Control 1/1(flag) -> flag/1
  Constant1/1 -> Model Predictive Control 1/18(R_in)

== system MPC_MG_freq_27072022/Sample /3to2 1 ==
  "Vabc_o " : Inport
  Add : Sum  Inputs=+++
  Constant : Constant  Value=exp(i*2*pi/3)
  Constant1 : Constant  Value=2/3
  Demux : Demux  Outputs=3
  Math Function : Math  Operator=square  SignedPower=on  SaturateOnIntegerOverflow=on
  Product : Product  RndMeth=Zero
  Product1 : Product  RndMeth=Zero
  Product2 : Product  RndMeth=Zero
  Vo : Outport  VectorParamsAs1DForOutWhenUnconnected=off
  wires:
  Add/1 -> Product/1
  Demux/1 -> Add/1
  Constant1/1 -> Product/2
  Product1/1 -> Add/2
  Constant/1 -> Product1/1, Math Function/1
  Demux/2 -> Product1/2
  Math Function/1 -> Product2/1
  Demux/3 -> Product2/2
  Product2/1 -> Add/3
  Product/1 -> Vo/1
  "Vabc_o "/1 -> Demux/1

== system MPC_MG_freq_27072022/Sample /3to2 2 ==
  "Iabc_o " : Inport
  Add : Sum  Inputs=+++
  Constant : Constant  Value=exp(i*2*pi/3)
  Constant1 : Constant  Value=2/3
  Demux : Demux  Outputs=3
  Math Function : Math  Operator=square  SignedPower=on  SaturateOnIntegerOverflow=on
  Product : Product  RndMeth=Zero
  Product1 : Product  RndMeth=Zero
  Product2 : Product  RndMeth=Zero
  Il : Outport  VectorParamsAs1DForOutWhenUnconnected=off
  wires:
  Add/1 -> Product/1
  Demux/1 -> Add/1
  Constant1/1 -> Product/2
  Product1/1 -> Add/2
  Constant/1 -> Product1/1, Math Function/1
  Demux/2 -> Product1/2
  Math Function/1 -> Product2/1
  Demux/3 -> Product2/2
  Product2/1 -> Add/3
  Product/1 -> Il/1
  "Iabc_o "/1 -> Demux/1

== system MPC_MG_freq_27072022/Sample /3to2 3 ==
  "single " : Inport
  "wt " : Inport  Port=2
  Add1 : Sum  Inputs=+++
  Constant2 : Constant  Value=2*pi/3
  Constant3 : Constant  Value=4*pi/3
  Constant4 : Constant  Value=exp(i*2*pi/3)
  Constant5 : Constant  Value=2/3
  Cos : Trigonometry  Operator=cos
  Cos1 : Trigonometry  Operator=cos
  Cos2 : Trigonometry  Operator=cos
  Math Function1 : Math  Operator=square  SignedPower=on  SaturateOnIntegerOverflow=on
  Product{3..8} (6 alike) : Product  RndMeth=Zero
  Scope : Scope  NumInputPorts=3
  Sum : Sum  Inputs=|++
  Sum1 : Sum  Inputs=|++
  threePhase : Outport  VectorParamsAs1DForOutWhenUnconnected=off
  wires:
  "single "/1 -> Product5/1, Product4/1, Product3/1
  Cos/1 -> Product3/2
  Constant2/1 -> Sum/2
  Sum/1 -> Cos1/1
  Cos1/1 -> Product4/2
  "wt "/1 -> Sum1/1, Sum/1, Cos/1
  Constant3/1 -> Sum1/2
  Sum1/1 -> Cos2/1
  Cos2/1 -> Product5/2
  Constant4/1 -> Product7/1, Math Function1/1
  Product7/1 -> Add1/2
  Add1/1 -> Product6/1
  Product8/1 -> Add1/3
  Product5/1 -> Scope/3, Product8/2
  Product6/1 -> threePhase/1
  Product3/1 -> Scope/1, Add1/1
  Constant5/1 -> Product6/2
  Product4/1 -> Scope/2, Product7/2
  Math Function1/1 -> Product8/1

== system MPC_MG_freq_27072022/Sample /Droop Controller ==
  note: Droop Controller
  note: Droop Input & Input Selection
  note: Virtual Impedance
  wni : Inport
  In2 : Inport  Port=2
  Q : Inport  Port=3
  P : Inport  Port=4
  Droop for secondary control2 : Subsystem
  Gain6 : Gain  Gain=LD_ref1
  High-Pass Filter : TransferFcn  Numerator=[1 0]  Denominator=w_c_high
  Sum : Sum  Inputs=|+-
  Sum1 : Sum  Inputs=|++
  Switch2 : Switch  Criteria=u2 > Threshold  Threshold=time_thresh
  V_nom1 : Constant  Value=V_nom
  w_nom1 : Constant  Value=w_nom
  w_nom2 : Constant  Value=0
  wt : Outport
  wo1 : Outport  Port=2
  Vref : Outport  Port=3
  wires:
  Sum1/1 -> Droop for secondary control2/2(w_nom)
  wni/1 -> Switch2/1
  Droop for secondary control2/3(wo) -> wo1/1
  [delay] -> Switch2/2
  V_nom1/1 -> Droop for secondary control2/3(V_nom)
  High-Pass Filter/1 -> Sum/2
  w_nom1/1 -> Sum1/2
  Sum/1 -> Vref/1
  Gain6/1 -> High-Pass Filter/1
  In2/1 -> Gain6/1
  Droop for secondary control2/1(Vref) -> Sum/1
  Q/1 -> Droop for secondary control2/4(Q)
  P/1 -> Droop for secondary control2/1(P)
  w_nom2/1 -> Switch2/3
  Switch2/1 -> Sum1/1
  Droop for secondary control2/2(wt) -> wt/1

== system MPC_MG_freq_27072022/Sample /Inverter Block ==
  "  " : Inport
  BL : Inport  Port=2
  Bus 1 : spsThreePhaseVIMeasurementLib/Three-Phase V-I Measurement  VoltageMeasurement=phase-to-ground  SetLabelV=off  LabelV=Vbus  Vpu=off  VpuLL=off  CurrentMeasurement=no  SetLabelI=off  LabelI=Ibus  Ipu=off  Pbase=100e6  Vbase=380  OutputType=Complex  PhasorSimulation=off  PSBequivalent=0
  DC Voltage Source1 : spsDCVoltageSourceLib/DC Voltage Source  Amplitude=Vdc  Measurements=None
  Ground : spsGroundLib/Ground  LConnTagsString=a
  Series RLC Branch : spsSeriesRLCBranchLib/Series RLC Branch  LConnTagsString=__new0  RConnTagsString=__new0  BranchType=RC  Resistance=30  Inductance=1e-3  SetiL0=off  InitialCurrent=0  Capacitance=80e-6  Setx0=off  InitialVoltage=0  Measurements=None
  Three-Phase Series RLC Branch : spsThreePhaseSeriesRLCBranchLib/Three-Phase Series RLC Branch  LConnTagsString=A|B|C  RConnTagsString=A|B|C  BranchType=RL  Resistance=R_f  Inductance=L_f  Capacitance=1e-6  Measurements=None
  Three-Phase Series RLC Branch1 : spsThreePhaseSeriesRLCBranchLib/Three-Phase Series RLC Branch  LConnTagsString=A|B|C  RConnTagsString=A|B|C  BranchType=RL  Resistance=R_in  Inductance=L_in  Capacitance=1e-6  Measurements=None
  Three-Phase Series RLC Branch2 : spsThreePhaseSeriesRLCBranchLib/Three-Phase Series RLC Branch  LConnTagsString=A|B|C  RConnTagsString=A|B|C  BranchType=C  Resistance=R_f  Inductance=1e-3  Capacitance=C_f  Measurements=None
  Three-Phase V-I Measurement : spsThreePhaseVIMeasurementLib/Three-Phase V-I Measurement  VoltageMeasurement=phase-to-ground  SetLabelV=off  LabelV=Vo1  Vpu=off  VpuLL=off  CurrentMeasurement=yes  SetLabelI=off  LabelI=Io1  Ipu=off  Pbase=100e6  Vbase=500e3  OutputType=Complex  PhasorSimulation=off  PSBequivalent=0
  Three-Phase V-I Measurement1 : spsThreePhaseVIMeasurementLib/Three-Phase V-I Measurement  VoltageMeasurement=phase-to-ground  SetLabelV=off  LabelV=Vl2  Vpu=off  VpuLL=off  CurrentMeasurement=yes  SetLabelI=off  LabelI=Il2  Ipu=off  Pbase=100e6  Vbase=500e3  OutputType=Complex  PhasorSimulation=off  PSBequivalent=0
  Two-Level Converter : spsTwoLevelConverterLib/Two-Level Converter  ModelType=Switching devices  Ron=1e-3  Rs=1e6  Cs=inf  Vforward=[0,0]  Ron_Diode=1e-3  Rs_Diode=1e6  Cs_Diode=inf  Vf_Diode=1e-3  Rs_CurrentSource=inf
      settings: SourceProductBaseCode=PS
  Conn1 : PMIOPort  Side=Left
  Conn2 : PMIOPort  Port=2  Side=Left
  Conn3 : PMIOPort  Port=3  Side=Left
  Vabc : Outport
  Iabc : Outport  Port=2
  Vabc1 : Outport  Port=3
  Vabc2 : Outport  Port=4
  wires:
  Three-Phase V-I Measurement1/1 -> Vabc1/1
  Three-Phase V-I Measurement/2 -> [Io]
  "  "/1 -> Two-Level Converter/1
  Bus 1/1 -> Vabc2/1
  Three-Phase V-I Measurement/1 -> Vabc/1
  Three-Phase V-I Measurement1/2 -> Iabc/1
  BL/1 -> Two-Level Converter/2
  connections:
  Three-Phase V-I Measurement/LConn2 -- Three-Phase Series RLC Branch1/RConn2
  Two-Level Converter/LConn2 -- Three-Phase V-I Measurement1/RConn2
  Bus 1/RConn3 -- Three-Phase Series RLC Branch1/LConn3
  Two-Level Converter/RConn2 -- Series RLC Branch/RConn1 -- DC Voltage Source1/LConn1
  Three-Phase Series RLC Branch/LConn2 -- Three-Phase Series RLC Branch2/LConn2 -- Three-Phase V-I Measurement/RConn2
  Two-Level Converter/RConn1 -- DC Voltage Source1/RConn1 -- Series RLC Branch/LConn1
  Three-Phase Series RLC Branch2/RConn3 -- Ground/LConn1 -- Three-Phase Series RLC Branch2/RConn1 -- Three-Phase Series RLC Branch2/RConn2
  Two-Level Converter/LConn3 -- Three-Phase V-I Measurement1/RConn3
  Conn1/RConn1 -- Bus 1/LConn1
  Three-Phase Series RLC Branch2/LConn3 -- Three-Phase Series RLC Branch/LConn3 -- Three-Phase V-I Measurement/RConn3
  Three-Phase Series RLC Branch1/RConn3 -- Three-Phase V-I Measurement/LConn3
  Three-Phase Series RLC Branch/RConn1 -- Three-Phase V-I Measurement1/LConn1
  Two-Level Converter/LConn1 -- Three-Phase V-I Measurement1/RConn1
  Three-Phase V-I Measurement/LConn1 -- Three-Phase Series RLC Branch1/RConn1
  Conn2/RConn1 -- Bus 1/LConn2
  Bus 1/RConn2 -- Three-Phase Series RLC Branch1/LConn2
  Bus 1/RConn1 -- Three-Phase Series RLC Branch1/LConn1
  Three-Phase Series RLC Branch2/LConn1 -- Three-Phase Series RLC Branch/LConn1 -- Three-Phase V-I Measurement/RConn1
  Three-Phase V-I Measurement1/LConn2 -- Three-Phase Series RLC Branch/RConn2
  Three-Phase Series RLC Branch/RConn3 -- Three-Phase V-I Measurement1/LConn3
  Conn3/RConn1 -- Bus 1/LConn3

== system MPC_MG_freq_27072022/Sample /PLL_1p1 ==
  v : Inport
  2pi : Constant  Value=2*pi
  Low-Pass Filter (Discrete or Continuous) : eeGeneralControl/Low-Pass Filter (Discrete or Continuous)  K=1  T=lo_co  B=inf  A=-inf  init_option=Inherited from block input  x0=0  Ts=-1
  PID Controller : slpidlib/PID Controller  Controller=PI  Form=Parallel  TimeDomain=Continuous-time  UseExternalTs=off  SampleTime=-1  IntegratorMethod=Forward Euler  FilterMethod=Forward Euler  ControllerParametersSource=internal  P=100.15925  I=9869  D=0  UseFilter=on  N=100  TunerSelectOption=Transfer Function Based (PID Tuner App)  InitialConditionSource=internal  InitialConditionForIntegrator=0  InitialConditionForFilter=0  DifferentiatorICPrevScaledInput=0  ExternalReset=none  TrackingMode=off  Kt=1  LimitOutput=off  SatLimitsSource=internal  UpperSaturationLimit=inf  LowerSaturationLimit=-inf  LinearizeAsGain=off  AntiWindupMode=none  Kb=1  POutMin=[]  POutMax=[]  IOutMin=[]  IOutMax=[]  DOutMin=[]  DOutMax=[]  NOutMin=[]  NOutMax=[]  SumOutMin=[]  SumOutMax=[]  SaturationOutMin=[]  SaturationOutMax=[]  PParamMin=[]  PParamMax=[]  IParamMin=[]  IParamMax=[]  DParamMin=[]  DParamMax=[]  NParamMin=[]  NParamMax=[]  KbParamMin=[]  KbParamMax=[]  KtParamMin=[]  KtParamMax=[]  KbOutMin=[]  KbOutMax=[]  KtOutMin=[]  KtOutMax=[]  IntegratorOutMin=[]  IntegratorOutMax=[]  FilterOutMin=[]  FilterOutMax=[]  SumI1OutMin=[]  SumI1OutMax=[]  SumI2OutMin=[]  SumI2OutMax=[]  SumI3OutMin=[]  SumI3OutMax=[]  SumI4OutMin=[]  SumI4OutMax=[]  SumDOutMin=[]  SumDOutMax=[]  DifferentiatorOutMin=[]  DifferentiatorOutMax=[]  FilterDiffOutCoefMin=[]  FilterDiffOutCoefMax=[]  ReciprocalOutMin=[]  ReciprocalOutMax=[]  SumDenOutMin=[]  SumDenOutMax=[]  SumNumOutMin=[]  SumNumOutMax=[]  DivideOutMin=[]  DivideOutMax=[]  UdiffTsProdOutMin=[]  UdiffTsProdOutMax=[]  NTsProdOutMin=[]  NTsProdOutMax=[]  UintegralTsProdOutMin=[]  UintegralTsProdOutMax=[]  UngainTsProdOutMin=[]  UngainTsProdOutMax=[]  IntegratorContinuousStateAttributes=''  IntegratorStateMustResolveToSignalObject=off  IntegratorRTWStateStorageClass=Auto  FilterContinuousStateAttributes=''  FilterStateMustResolveToSignalObject=off  FilterRTWStateStorageClass=Auto  ParallelPVariant=InternalParameters  IdealPVariant=Disabled  IVariant=InternalParameters  DVariant=Disabled  IntegratorVariant=Continuous  SatVariant=Disabled  AWVariant=Passthrough  PCopyVariant=Disabled  TRVariant=Disabled  FdbkBlocksVariant=Forward  IdealPFdbkVariant=Disabled  SatFdbkVariant=Disabled  DerivativeFilterVariant=Disabled  NVariant=Disabled  NCopyVariant=Disabled_SignalSpec  FilterICVariant=Disabled  IntegratorICVariant=InternalICs  ExternalResetVariant=Disabled  TRSumVariant=Passthrough  SumFdbkVariant=Disabled  SumVariant=Sum_PI  TsampFilterVariant=InternalTs  TsampNgainVariant=Passthrough  TsampIntegralVariant=Passthrough  ExternalSaturationOutDataTypeStr=Inherit: Same as second input
  Reset1 : RelationalOperator  OutDataTypeStr=boolean  RndMeth=Nearest
  Sqrt : Sqrt  SaturateOnIntegerOverflow=on
  Square : Math  Operator=square  SaturateOnIntegerOverflow=on
  Square1 : Math  Operator=square  SaturateOnIntegerOverflow=on
  Sum : Sum  Inputs=|++
  Sum1 : Sum  Inputs=|++
  TienXuly : Subsystem  mask{k=0.5, fc1=50, fc2=10}
      mask prompts: k "he so k"; fc1 "Tan so cat cua bo loc bac 2"; fc2 "Tan so cat cua bo loc thong thap"
  Tinhtheta : Integrator  ExternalReset=rising  UpperSaturationLimit=2*pi
  apha-beta=>dq : Subsystem
  wff : Constant  Value=50*2*pi
  v_dq : Outport
  omega : Outport  Port=2
  wires:
  PID Controller/1 -> Sum1/1
  v/1 -> TienXuly/1(v)
  Tinhtheta/1 -> apha-beta=>dq/1(Theta), Reset1/1
  TienXuly/2(v'q) -> apha-beta=>dq/3(Ubeta)
  apha-beta=>dq/1(vq) -> Square1/1, PID Controller/1
  TienXuly/1(v') -> apha-beta=>dq/2(Uapha)
  2pi/1 -> Reset1/2
  wff/1 -> Sum1/2
  Reset1/1 -> Tinhtheta/2
  apha-beta=>dq/2(vd) -> Square/1
  Square/1 -> Sum/1
  Square1/1 -> Sum/2
  Sum/1 -> Sqrt/1
  Sqrt/1 -> v_dq/1
  Sum1/1 -> Low-Pass Filter (Discrete or Continuous)/1, Tinhtheta/1  "P"
  Low-Pass Filter (Discrete or Continuous)/1 -> omega/1  "P"

== system MPC_MG_freq_27072022/Sample /PLL_1p2 ==
  v : Inport
  2pi : Constant  Value=2*pi
  Low-Pass Filter (Discrete or Continuous) : eeGeneralControl/Low-Pass Filter (Discrete or Continuous)  K=1  T=lo_co  B=inf  A=-inf  init_option=Inherited from block input  x0=0  Ts=-1
  PID Controller : slpidlib/PID Controller  Controller=PI  Form=Parallel  TimeDomain=Continuous-time  UseExternalTs=off  SampleTime=-1  IntegratorMethod=Forward Euler  FilterMethod=Forward Euler  ControllerParametersSource=internal  P=100.15925  I=9869  D=0  UseFilter=on  N=100  TunerSelectOption=Transfer Function Based (PID Tuner App)  InitialConditionSource=internal  InitialConditionForIntegrator=0  InitialConditionForFilter=0  DifferentiatorICPrevScaledInput=0  ExternalReset=none  TrackingMode=off  Kt=1  LimitOutput=off  SatLimitsSource=internal  UpperSaturationLimit=inf  LowerSaturationLimit=-inf  LinearizeAsGain=off  AntiWindupMode=none  Kb=1  POutMin=[]  POutMax=[]  IOutMin=[]  IOutMax=[]  DOutMin=[]  DOutMax=[]  NOutMin=[]  NOutMax=[]  SumOutMin=[]  SumOutMax=[]  SaturationOutMin=[]  SaturationOutMax=[]  PParamMin=[]  PParamMax=[]  IParamMin=[]  IParamMax=[]  DParamMin=[]  DParamMax=[]  NParamMin=[]  NParamMax=[]  KbParamMin=[]  KbParamMax=[]  KtParamMin=[]  KtParamMax=[]  KbOutMin=[]  KbOutMax=[]  KtOutMin=[]  KtOutMax=[]  IntegratorOutMin=[]  IntegratorOutMax=[]  FilterOutMin=[]  FilterOutMax=[]  SumI1OutMin=[]  SumI1OutMax=[]  SumI2OutMin=[]  SumI2OutMax=[]  SumI3OutMin=[]  SumI3OutMax=[]  SumI4OutMin=[]  SumI4OutMax=[]  SumDOutMin=[]  SumDOutMax=[]  DifferentiatorOutMin=[]  DifferentiatorOutMax=[]  FilterDiffOutCoefMin=[]  FilterDiffOutCoefMax=[]  ReciprocalOutMin=[]  ReciprocalOutMax=[]  SumDenOutMin=[]  SumDenOutMax=[]  SumNumOutMin=[]  SumNumOutMax=[]  DivideOutMin=[]  DivideOutMax=[]  UdiffTsProdOutMin=[]  UdiffTsProdOutMax=[]  NTsProdOutMin=[]  NTsProdOutMax=[]  UintegralTsProdOutMin=[]  UintegralTsProdOutMax=[]  UngainTsProdOutMin=[]  UngainTsProdOutMax=[]  IntegratorContinuousStateAttributes=''  IntegratorStateMustResolveToSignalObject=off  IntegratorRTWStateStorageClass=Auto  FilterContinuousStateAttributes=''  FilterStateMustResolveToSignalObject=off  FilterRTWStateStorageClass=Auto  ParallelPVariant=InternalParameters  IdealPVariant=Disabled  IVariant=InternalParameters  DVariant=Disabled  IntegratorVariant=Continuous  SatVariant=Disabled  AWVariant=Passthrough  PCopyVariant=Disabled  TRVariant=Disabled  FdbkBlocksVariant=Forward  IdealPFdbkVariant=Disabled  SatFdbkVariant=Disabled  DerivativeFilterVariant=Disabled  NVariant=Disabled  NCopyVariant=Disabled_SignalSpec  FilterICVariant=Disabled  IntegratorICVariant=InternalICs  ExternalResetVariant=Disabled  TRSumVariant=Passthrough  SumFdbkVariant=Disabled  SumVariant=Sum_PI  TsampFilterVariant=InternalTs  TsampNgainVariant=Passthrough  TsampIntegralVariant=Passthrough  ExternalSaturationOutDataTypeStr=Inherit: Same as second input
  Reset1 : RelationalOperator  OutDataTypeStr=boolean  RndMeth=Nearest
  Scope : Scope
  Sqrt : Sqrt  SaturateOnIntegerOverflow=on
  Square : Math  Operator=square  SaturateOnIntegerOverflow=on
  Square1 : Math  Operator=square  SaturateOnIntegerOverflow=on
  Sum : Sum  Inputs=|++
  Sum1 : Sum  Inputs=|++
  TienXuly : Subsystem  mask{k=0.5, fc1=50, fc2=10}
      mask prompts: k "he so k"; fc1 "Tan so cat cua bo loc bac 2"; fc2 "Tan so cat cua bo loc thong thap"
  Tinhtheta : Integrator  ExternalReset=rising  UpperSaturationLimit=2*pi
  apha-beta=>dq : Subsystem
  wff : Constant  Value=50*2*pi
  v_dq : Outport
  omega : Outport  Port=2
  wires:
  PID Controller/1 -> Sum1/1
  v/1 -> TienXuly/1(v)
  Tinhtheta/1 -> apha-beta=>dq/1(Theta), Reset1/1
  TienXuly/2(v'q) -> apha-beta=>dq/3(Ubeta)
  apha-beta=>dq/1(vq) -> Square1/1, PID Controller/1
  TienXuly/1(v') -> apha-beta=>dq/2(Uapha)
  2pi/1 -> Reset1/2
  wff/1 -> Sum1/2
  Reset1/1 -> Tinhtheta/2
  apha-beta=>dq/2(vd) -> Square/1
  Square/1 -> Sum/1
  Square1/1 -> Sum/2
  Sum/1 -> Sqrt/1
  Sqrt/1 -> v_dq/1
  Sum1/1 -> Low-Pass Filter (Discrete or Continuous)/1, Tinhtheta/1  "P"
  Low-Pass Filter (Discrete or Continuous)/1 -> Scope/1, omega/1  "P"
